simulink model "tcp_bbr"  (R2015b)
settings: Solver=FixedStepAuto  StartTime=0.0  StopTime=6  FixedStep=0.001  RelTol=1e-3
settings Model: Creator=lenovo  LastModifiedBy=lenovo

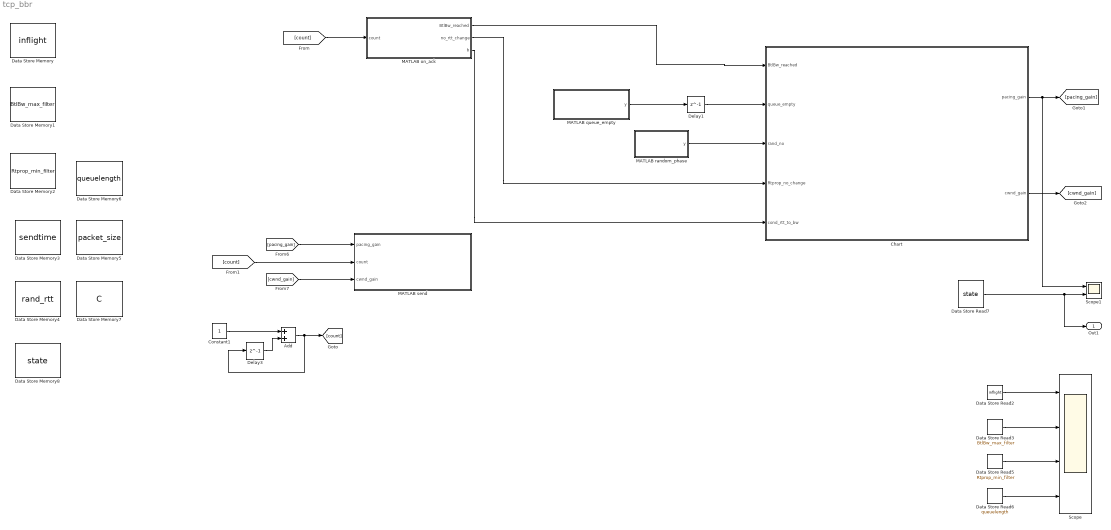
== system tcp_bbr ==
  Add : Sum
  Chart : Stateflow chart  TreatAsAtomicUnit=on
  Constant1 : Constant
  Data Store Memory : DataStoreMemory  DataStoreName=inflight  ReadBeforeWriteMsg=warning  WriteAfterWriteMsg=warning  WriteAfterReadMsg=warning  OutDataTypeStr=double
  Data Store Memory1 : DataStoreMemory  DataStoreName=BtlBw_max_filter  ReadBeforeWriteMsg=warning  WriteAfterWriteMsg=warning  WriteAfterReadMsg=warning  OutDataTypeStr=double
  Data Store Memory2 : DataStoreMemory  DataStoreName=Rtprop_min_filter  ReadBeforeWriteMsg=warning  WriteAfterWriteMsg=warning  WriteAfterReadMsg=warning  InitialValue=400  OutDataTypeStr=double
  Data Store Memory3 : DataStoreMemory  DataStoreName=sendtime  ReadBeforeWriteMsg=warning  WriteAfterWriteMsg=warning  WriteAfterReadMsg=warning  InitialValue=zeros(1,6000)  OutDataTypeStr=double
  Data Store Memory4 : DataStoreMemory  DataStoreName=rand_rtt  ReadBeforeWriteMsg=warning  WriteAfterWriteMsg=warning  WriteAfterReadMsg=warning  InitialValue=zeros(1,6000)  OutDataTypeStr=double
  Data Store Memory5 : DataStoreMemory  DataStoreName=packet_size  ReadBeforeWriteMsg=warning  WriteAfterWriteMsg=warning  WriteAfterReadMsg=warning  InitialValue=8192  VectorParams1D=off  OutDataTypeStr=double
  Data Store Memory6 : DataStoreMemory  DataStoreName=queuelength  ReadBeforeWriteMsg=warning  WriteAfterWriteMsg=warning  WriteAfterReadMsg=warning  VectorParams1D=off  OutDataTypeStr=double
  Data Store Memory7 : DataStoreMemory  DataStoreName=C  ReadBeforeWriteMsg=warning  WriteAfterWriteMsg=warning  WriteAfterReadMsg=warning  InitialValue=128  VectorParams1D=off  OutDataTypeStr=double
  Data Store Memory8 : DataStoreMemory  DataStoreName=state  ReadBeforeWriteMsg=warning  WriteAfterWriteMsg=warning  WriteAfterReadMsg=warning  InitialValue=1  VectorParams1D=off  OutDataTypeStr=double
  Data Store Read2 : DataStoreRead  DataStoreName=inflight
  Data Store Read3 : DataStoreRead  DataStoreName=BtlBw_max_filter
  Data Store Read5 : DataStoreRead  DataStoreName=Rtprop_min_filter
  Data Store Read6 : DataStoreRead  DataStoreName=queuelength
  Data Store Read7 : DataStoreRead  DataStoreName=state
  Delay1 : Delay  DelayLength=1  InitialCondition=0
  Delay3 : Delay  DelayLength=1  InitialCondition=0
  MATLAB on_ack : MATLAB Function  TreatAsAtomicUnit=on
  MATLAB queue_empty : MATLAB Function  TreatAsAtomicUnit=on
  MATLAB random_phase : MATLAB Function  TreatAsAtomicUnit=on
  MATLAB send : MATLAB Function  TreatAsAtomicUnit=on
  Scope : Scope  NumInputPorts=4
  Scope1 : Scope  NumInputPorts=2
  Out1 : Outport
  wires:
  MATLAB queue_empty/1(y) -> Delay1/1
  MATLAB random_phase/1(y) -> Chart/3(rand_no)
  Constant1/1 -> Add/1
  Delay3/1 -> Add/2
  Add/1 -> Delay3/1, [count]
  Chart/1(pacing_gain) -> Scope1/1, [pacing_gain]
  Chart/2(cwnd_gain) -> [cwnd_gain]
  [count] -> MATLAB on_ack/1(count)
  [count] -> MATLAB send/2(count)
  [pacing_gain] -> MATLAB send/1(pacing_gain)
  [cwnd_gain] -> MATLAB send/3(cwnd_gain)
  MATLAB on_ack/1(BtlBw_reached) -> Chart/1(BtlBw_reached)
  MATLAB on_ack/2(no_rtt_change) -> Chart/4(Rtprop_no_change)
  Data Store Read2/1 -> Scope/1
  Data Store Read3/1 -> Scope/2
  Data Store Read5/1 -> Scope/3
  Data Store Read6/1 -> Scope/4
  Data Store Read7/1 -> Out1/1, Scope1/2
  MATLAB on_ack/3(b) -> Chart/5(cond_rtt_to_bw)
  Delay1/1 -> Chart/2(queue_empty)

== matlab function tcp_bbr/MATLAB queue_empty ==
  data: y output; inflight data_store_memory; queuelength data_store_memory; C data_store_memory; rand_rtt data_store_memory; BtlBw_max_filter data_store_memory; Rtprop_min_filter data_store_memory; packet_size data_store_memory
function y = queue_isempty()
%#codegen
global inflight;
global BtlBw_max_filter;
global Rtprop_min_filter;
global packet_size;

global queuelength;
persistent packet_no;
global rand_rtt;
global C;

if(isempty(packet_no))
    packet_no = 1;
end

if(rand_rtt(packet_no)~=0)
    queuelength = inflight - (C*rand_rtt(packet_no)/1000);
    if queuelength < 0
        queuelength = 0;
    end
    packet_no = packet_no+1;
end


if (inflight * packet_size <= BtlBw_max_filter * Rtprop_min_filter/1000)
    y = true;
else
    y = false;
end

== stateflow chart tcp_bbr/Chart ==
  state DRAIN
    entry:
    state = 2
    pacing_gain = 1/2.89
    cwnd_gain = 2.89
  state STARTUP
    entry:
    state = 1
    pacing_gain = 2.89
    cwnd_gain = 2.89
  state ProbeBW
    entry:
    state= 3
    cwnd_gain = 2.89
    state entry_1
      entry: pacing_gain = 1.25
    state entry_
      entry:  pacing_gain = 0.75
    state entry_2
      entry: pacing_gain = 1
    (default) -> (junction 15) : [rand_no]
    (junction 15) -> entry_1 [order 1] : [rand_no<3]
    (junction 15) -> entry_2 [order 2] : [rand_no>=3]
    entry_1 -> entry_
    entry_2 -> entry_1 : after(6,tick)
    entry_ -> entry_2
  state ProbeRTT
    entry:
    state = 4
    pacing_gain = 1
    cwnd_gain = 1
  (default) -> STARTUP
  STARTUP -> DRAIN : [BtlBw_reached]
  DRAIN -> ProbeBW : [queue_empty]
  ProbeRTT -> STARTUP [order 1] : [after(200,tick)&&~cond_rtt_to_bw]
  ProbeRTT -> ProbeBW [order 2] : [after(200,tick)&&cond_rtt_to_bw]
  ProbeBW -> ProbeRTT : [Rtprop_no_change]
  data: BtlBw_reached input boolean; queue_empty input boolean; rand_no input; pacing_gain output double; cwnd_gain output double; Rtprop_no_change input boolean; cond_rtt_to_bw input boolean; state data_store_memory

== matlab function tcp_bbr/MATLAB random_phase ==
  data: y output
function y = random_phase()
%#codegen
rng(0,'twister')
y = randi([1 8],1,1);
end

== matlab function tcp_bbr/MATLAB on_ack ==
  data: sendtime data_store_memory; count input; BtlBw_max_filter data_store_memory; Rtprop_min_filter data_store_memory; rand_rtt data_store_memory; BtlBw_reached output; no_rtt_change output; inflight data_store_memory; packet_size data_store_memory; b output
function [BtlBw_reached,no_rtt_change,b]= on_ACK(count)
%#codegen

persistent packet_no;
persistent count_t;
persistent delivery_rate;


global inflight;
global BtlBw_max_filter;
global Rtprop_min_filter;
global sendtime;
global rand_rtt;
global packet_size;


if (isempty(count_t))
    count_t = 0;
end


if (isempty(delivery_rate))
    delivery_rate = 0;
end


if (isempty(packet_no))
    packet_no = 1;
end



BtlBw_reached = false;
no_rtt_change = false;


if ((count-1) >= (sendtime(packet_no)+rand_rtt(packet_no))&& rand_rtt(packet_no)~=0)
    temp = Rtprop_min_filter;
    Rtprop_min_filter = min(Rtprop_min_filter,rand_rtt(packet_no));
    delta = abs(temp - Rtprop_min_filter);
    percent_delta = delta/temp;
    
    if(percent_delta <= 0.25)
        no_rtt_change = true;
    else
        no_rtt_change = false;
    end
    
    %%BtlBw
    
    delivery_rate = inflight*packet_size*1000 / rand_rtt(packet_no);
    
    temp = BtlBw_max_filter;
    BtlBw_max_filter = max(delivery_rate,BtlBw_max_filter);
    delta = abs(temp - BtlBw_max_filter);
    percent_delta = delta/temp;
    
    if(percent_delta <= 0.25)
        count_t = count_t + 1;
        if( count_t == 3)
            BtlBw_reached = true;
            count_t = 0;
        else
            BtlBw_reached = false;
        end
    else
        count_t = 0;
    end
    
    packet_no = packet_no+1;
    inflight = inflight - 1;
end

if(delivery_rate < BtlBw_max_filter)
    b = false;
else
    b = true;
end
end

== matlab function tcp_bbr/MATLAB send ==
  data: pacing_gain input; sendtime data_store_memory; count input; BtlBw_max_filter data_store_memory; inflight data_store_memory; rand_rtt data_store_memory; Rtprop_min_filter data_store_memory; cwnd_gain input; packet_size data_store_memory; C data_store_memory; queuelength data_store_memory; state data_store_memory
function send(pacing_gain,count,cwnd_gain)
%#codegen

persistent sent_packet_no;

global inflight;
global BtlBw_max_filter;
global Rtprop_min_filter;
global sendtime;
global rand_rtt;
global packet_size;
global C;
global queuelength;
global state;

if (isempty(sent_packet_no))
    sent_packet_no = 1;
end

bdp = BtlBw_max_filter*Rtprop_min_filter/1000;
if(inflight*packet_size>cwnd_gain*bdp)
    return    
end

if ((count-1) >= sendtime(sent_packet_no))
    rand_rtt(sent_packet_no) = 100 + (queuelength*1000)/C;  %10ms propagation delay
    
    if(BtlBw_max_filter~=0)
        sendtime(sent_packet_no+1) = round(count - 1 + (packet_size *1000 / (pacing_gain*BtlBw_max_filter)));
    else
        sendtime(sent_packet_no+1) = count;
    end
    
    inflight = inflight + 1;
    
    if(state==4)
        inflight = inflight+3;
        rand_rtt(sent_packet_no+1) = 100 + (queuelength*1000)/C;
        rand_rtt(sent_packet_no+2) = 100 + (queuelength*1000)/C;
        rand_rtt(sent_packet_no+3) = 100 + (queuelength*1000)/C;
        sent_packet_no = sent_packet_no + 3;
    end

    sent_packet_no = sent_packet_no + 1;
end

end
